simulink model "cruiseControlModel2018b"  (R2022b)
settings: Solver=VariableStepAuto  StartTime=0.0  StopTime=10.0  RelTol=1e-3
values from neighbouring files (symbols this model uses):
  a = 0.03    [cruiseControl_Init.m]
  b = 0.001    [cruiseControl_Init.m]
  F_FF = 0.5*rho*Cd*Af*V_FF.^2+(a+b*V_FF)*g*M_veh    [cruiseControl_Init.m]
  g = 9.81    [cruiseControl_Init.m]
  gradeFlag = 1    [cruiseControl_Init.m]
  ki = 150    [cruiseControl_Init.m]
  Kp = 1000    [cruiseControl_Init.m]
  M_tot = M_veh + M_eq    (= 2600)    [cruiseControl_Init.m]
  M_veh = 2400    [cruiseControl_Init.m]
  V0 = 25.5    [cruiseControl_Init.m]
  V1 = 2.2352    [cruiseControl_Init.m]
  V2 = 2.2352*2    (= 4.4704)    [cruiseControl_Init.m]
  V3 = 2.2352    [cruiseControl_Init.m]
  V4 = -2.2352*3    (= -6.7056)    [cruiseControl_Init.m]
  V5 = 2.2352    [cruiseControl_Init.m]
  V6 = 2.2352    [cruiseControl_Init.m]
  V7 = -2.2352    [cruiseControl_Init.m]
  V_FF = 0:5:40    [cruiseControl_Init.m]
undefined symbols (not defined in the file or in its folder): roadGrade
settings Model: LastModifiedBy=77dal
settings OptimizationCC: BlockReduction=off  BooleanDataType=off
settings DebuggingCC: SaveWithParameterizedLinksMsg=none  UnderspecifiedInitializationDetection=Classic  MergeDetectMultiDrivingBlocksExec=none  SignalResolutionControl=TryResolveAllWithWarning
settings HardwareCC: TargetUnknown=on
settings ModelReferenceCC: PropagateSignalLabelsOutOfModel=off

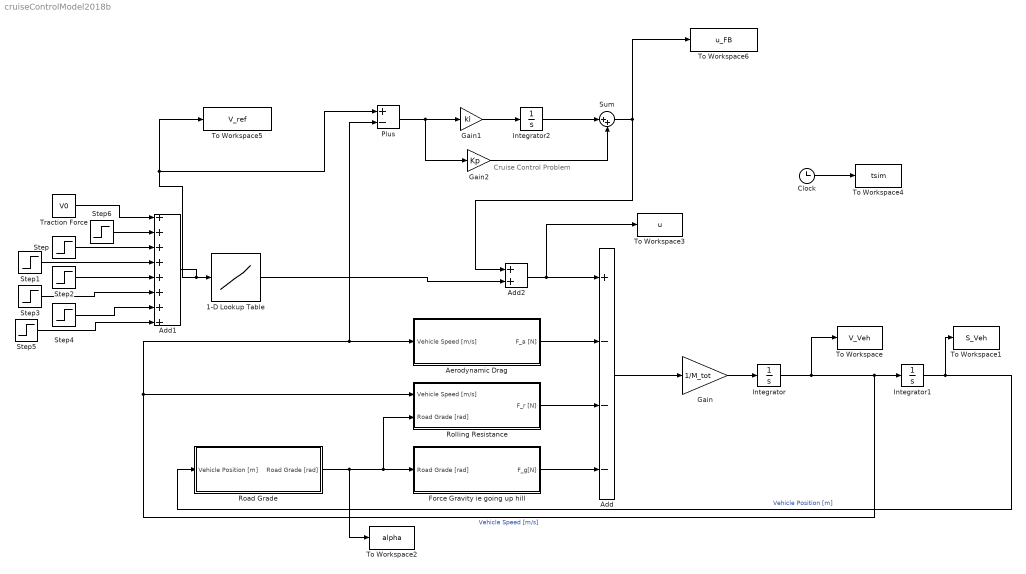
== system cruiseControlModel2018b ==
  note: Cruise Control Problem
  1-D Lookup Table : Lookup_n-D  NumberOfTableDimensions=1  BreakpointsForDimension1=V_FF  Table=F_FF  InternalRulePriority=Speed  RndMeth=Simplest
  Add : Sum  Inputs=+---
  Add1 : Sum  Inputs=++++++++
  Add2 : Sum
  Aerodynamic Drag : Subsystem
  Clock : Clock
  Force Gravity ie going up hill : Subsystem
  Gain : Gain  Gain=1/M_tot
  Gain1 : Gain  Gain=ki
  Gain2 : Gain  Gain=Kp
  Integrator : Integrator  InitialCondition=V0
  Integrator1 : Integrator
  Integrator2 : Integrator
  Plus : Sum  Inputs=+-
  Road Grade : Subsystem
  Rolling Resistance : Subsystem
  Step : Step  Before=100  After=V2  SampleTime=0
  Step1 : Step  Time=150  After=V3  SampleTime=0
  Step2 : Step  Time=250  After=V4  SampleTime=0
  Step3 : Step  Time=400  After=V5  SampleTime=0
  Step4 : Step  Time=450  After=V6  SampleTime=0
  Step5 : Step  Time=550  After=V7  SampleTime=0
  Step6 : Step  Time=50  After=V1  SampleTime=0
  Sum : Sum  Inputs=|++
  To Workspace : ToWorkspace  VariableName=V_Veh  SampleTime=-1
  To Workspace1 : ToWorkspace  VariableName=S_Veh  SampleTime=-1
  To Workspace2 : ToWorkspace  VariableName=alpha  SampleTime=-1
  To Workspace3 : ToWorkspace  VariableName=u  SampleTime=-1
  To Workspace4 : ToWorkspace  VariableName=tsim  SampleTime=-1
  To Workspace5 : ToWorkspace  VariableName=V_ref  SampleTime=-1
  To Workspace6 : ToWorkspace  VariableName=u_FB  SampleTime=-1
  Traction Force : Constant  Value=V0
  wires:
  Gain/1 -> Integrator/1
  Add/1 -> Gain/1
  Integrator/1 -> To Workspace/1, Plus/2, Aerodynamic Drag/1(Vehicle Speed [m/s]), Rolling Resistance/1(Vehicle Speed [m/s]), Integrator1/1  "Vehicle Speed [m/s]"
  Integrator1/1 -> To Workspace1/1, Road Grade/1(Vehicle Position [m])  "Vehicle Position [m]"
  Road Grade/1(Road Grade [rad]) -> Rolling Resistance/2(Road Grade [rad]), Force Gravity ie going up hill/1(Road Grade [rad]), To Workspace2/1
  Aerodynamic Drag/1(F_a [N]) -> Add/2
  Rolling Resistance/1(F_r [N]) -> Add/3
  Force Gravity ie going up hill/1(F_g[N]) -> Add/4
  Clock/1 -> To Workspace4/1
  Traction Force/1 -> Add1/1
  Add1/1 -> To Workspace5/1, Plus/1, 1-D Lookup Table/1
  Gain1/1 -> Integrator2/1
  Integrator2/1 -> Sum/1
  Gain2/1 -> Sum/2
  Plus/1 -> Gain2/1, Gain1/1
  Sum/1 -> Add2/1, To Workspace6/1
  1-D Lookup Table/1 -> Add2/2
  Add2/1 -> To Workspace3/1, Add/1
  Step/1 -> Add1/3
  Step1/1 -> Add1/4
  Step2/1 -> Add1/5
  Step3/1 -> Add1/6
  Step4/1 -> Add1/7
  Step5/1 -> Add1/8
  Step6/1 -> Add1/2

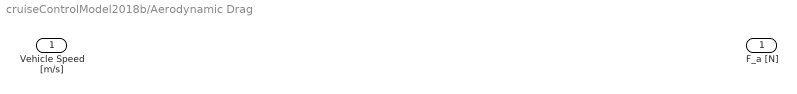
== system cruiseControlModel2018b/Aerodynamic Drag ==
  Vehicle Speed [m/s] : Inport
  F_a [N] : Outport

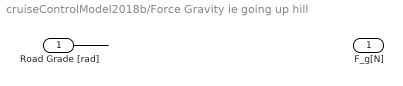
== system cruiseControlModel2018b/Force Gravity ie going up hill ==
  Road Grade [rad] : Inport
  F_g[N] : Outport
  wires:
  Road Grade [rad]/1 -> ?

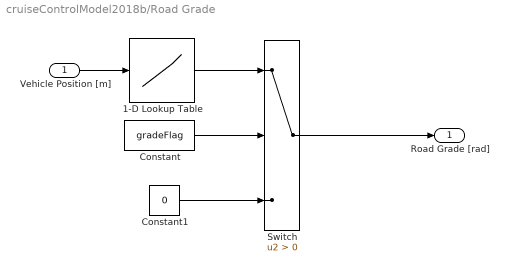
== system cruiseControlModel2018b/Road Grade ==
  Vehicle Position [m] : Inport
  1-D Lookup Table : Lookup_n-D  NumberOfTableDimensions=1  BreakpointsForDimension1=roadGrade.position  Table=roadGrade.alpha  InternalRulePriority=Speed  RndMeth=Simplest
  Constant : Constant  Value=gradeFlag
  Constant1 : Constant  Value=0
  Switch : Switch  Criteria=u2 > Threshold  SaturateOnIntegerOverflow=off  InputSameDT=off
  Road Grade [rad] : Outport
  wires:
  Vehicle Position [m]/1 -> 1-D Lookup Table/1
  1-D Lookup Table/1 -> Switch/1
  Constant/1 -> Switch/2
  Constant1/1 -> Switch/3
  Switch/1 -> Road Grade [rad]/1

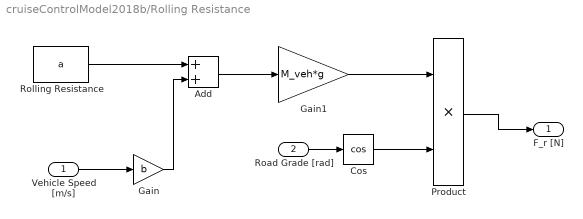
== system cruiseControlModel2018b/Rolling Resistance ==
  Vehicle Speed [m/s] : Inport
  Road Grade [rad] : Inport  Port=2
  Add : Sum
  Cos : Trigonometry  Operator=cos
  Gain : Gain  Gain=b
  Gain1 : Gain  Gain=M_veh*g
  Product : Product
  Rolling Resistance : Constant  Value=a
  F_r [N] : Outport
  wires:
  Rolling Resistance/1 -> Add/1
  Vehicle Speed [m/s]/1 -> Gain/1
  Gain/1 -> Add/2
  Add/1 -> Gain1/1
  Road Grade [rad]/1 -> Cos/1
  Product/1 -> F_r [N]/1
  Gain1/1 -> Product/1
  Cos/1 -> Product/2
